simulink model "Model_plane5Old_vers"  (R2021a)
settings: Solver=VariableStepAuto  StartTime=0.0  StopTime=200  RelTol=1e-3
model workspace (MAT data in the model file):
  Alfa = [-2 4 10 16]
  Alfa_table = [-4 0 5 10 20]
  Alfa_y = [-4 6 8 9 10 12 14]
  Cxa_table = [0.03434  0.0358  0.04274; 0.02598  0.0252  0.0262; 0.04151  0.0505  0.0883; 0.122  0.1649  0.2341; 0.502  0.538  0.666]
  Cy_DB = [0.01242 0.01286 0.01457]
  Cy_fi = [0.00623 0.00643 0.00626]
  Cya = [-0.276  -0.33  -0.39; 0.859  0.991  0.82; 1.085  1.211  1.1; 1.2  1.275  1.031; 1.296  1.29  1.018; 1.45  1.178  1.043; 1.461  1.163  1.081]
  H = [339 3256 4060 8000 12000]
  H_table = [0 2000 4000 6000 8000 10000]
  M_C = [0.4 0.6 0.82]
  M_mz = [0.2 0.4 0.6 0.8]
  M_mz2 = [0.4 0.7 0.85]
  M_table = [0.4 0.7 0.82]
  M_y = [0.4 0.7 0.82]
  P = [50000 40000 32000 25600 20480]
  a_table = [340.3 339.5 338.8 338 337.2 336.4]
  mz_DB = [-0.035 -0.0358 -0.037 -0.0377]
  mz_alfa = [-0.0282 -0.0282 -0.0289 -0.0404]
  mz_alfa2 = [-8.163  -8.762  -9.714; -8.163  -8.762  -9.583; -7.975  -7.991  -7.868; -6.514  -6.413  -6.732]
  mz_fi = [-0.0695 -0.0714 -0.0739 -0.0832]
  mz_omz = [-23.768  -25.3  -28.284; -23.768  -25.3  -27.903; -23.222  -22.6  -23.32; -18.967  -18.52  -19.601]
  out = Simulink.SimulationOutput
  out.Data.tout = [0 1.67688873362e-06 9.33181354111e-06 4.76064375786e-05 0.000238979557766 0.0011958451587 0.00598017316339 0.0291858115735 0.107609227908 0.294605508218 0.534390352194 0.619831316604 ... (6422 elements, 6422x1)]
  out.Metadata = Simulink.SimulationMetadata
  out.Metadata.ModelInfo.ModelName = 'Model_plane2'
  out.Metadata.ModelInfo.ModelVersion = '1.11'
  out.Metadata.ModelInfo.ModelFilePath = 'C:\Users\Анастасия\Универ\Mathlab\Модель самолёта\Model_plane2.slx'
  out.Metadata.ModelInfo.UserID = 'Анастасия'
  out.Metadata.ModelInfo.MachineName = 'DESKTOP-OE36224'
  out.Metadata.ModelInfo.Platform = 'PCWIN64'
  out.Metadata.ModelInfo.ModelStructuralChecksum = [329193822; 1830100004; 2373400892; 4162968501]
  out.Metadata.ModelInfo.SimulationMode = 'normal'
  out.Metadata.ModelInfo.StartTime = 0
  out.Metadata.ModelInfo.StopTime = 100
  out.Metadata.ModelInfo.SolverInfo.Type = 'Variable-Step'
  out.Metadata.ModelInfo.SolverInfo.Solver = 'ode45'
  out.Metadata.ModelInfo.SolverInfo.MaxStepSize = 2
  out.Metadata.ModelInfo.SimulinkVersion.Name = 'Simulink'
  out.Metadata.ModelInfo.SimulinkVersion.Version = '24.1'
  out.Metadata.ModelInfo.SimulinkVersion.Release = '(R2024a)'
  out.Metadata.ModelInfo.SimulinkVersion.Date = '19-Nov-2023'
  out.Metadata.ModelInfo.LoggingInfo.LoggingToFile = 'off'
  out.Metadata.TimingInfo.WallClockTimestampStart = '2025-02-14 11:01:22'
  out.Metadata.TimingInfo.WallClockTimestampStop = '2025-02-14 11:01:24'
  out.Metadata.TimingInfo.InitializationElapsedWallTime = 1.1990057
  out.Metadata.TimingInfo.ExecutionElapsedWallTime = 1.0786509
  out.Metadata.TimingInfo.TerminationElapsedWallTime = 0.0112241
  out.Metadata.TimingInfo.TotalElapsedWallTime = 2.2888807
  out.Metadata.TimingInfo.ProfilerData = 'Profiler is not enabled'
  out.Metadata.ExecutionInfo.StopEvent = 'ReachedStopTime'
  out.Metadata.ExecutionInfo.StopEventSource = []
  out.Metadata.ExecutionInfo.StopEventDescription = 'Reached stop time of 100'
  out.Metadata.ExecutionInfo.ErrorDiagnostic = []
  out.Metadata.ExecutionInfo.WarningDiagnostics.Diagnostic = MSLDiagnostic
  out.Metadata.ExecutionInfo.WarningDiagnostics.Diagnostic.identifier = 'Simulink:blocks:DivideByZero'
  out.Metadata.ExecutionInfo.WarningDiagnostics.Diagnostic.message = 'Division by zero in ''<a href="matlab:open_and_hilite_hyperlink (''Model_plane2/Уравнения продольного движения в связанной системе координат/Блок расчёта угла атаки Alfa/Divide'',''error'')">Model_plane2/Уравнения продольного движения в связанной системе координат/Блок расчёта угла атаки Alfa/Divide</a>'''
  out.Metadata.ExecutionInfo.WarningDiagnostics.Diagnostic.paths = {'Model_plane2/Уравнения продольного движения в связанной системе координат/Блок расчёта угла атаки Alfa/Divide'}
  out.Metadata.ExecutionInfo.WarningDiagnostics.Diagnostic.arguments = {'Model_plane2/Уравнения продольного движения в связанной системе координат/Блок расчёта угла атаки Alfa/Divide'}
  out.Metadata.ExecutionInfo.WarningDiagnostics.Diagnostic.stack = struct([])
  out.Metadata.ExecutionInfo.WarningDiagnostics.Diagnostic.actionProp = '22 serialization::archive 19 0 0 0  0 1 0 0 1 1 0 0 0 0 0 1 47 SL_SERVICES:utils:EMBEDDED____ACTION____WRAPPER 2 2 0 0 183 0 109 97 116 108 97 98 58 83 105 109 117 108 105 110 107 46 83 117 112 112 114 101 115 115 101 100 68 105 97 103 110 111 115 116 105 99 40 123 39 77 111 100 101 108 95 112 108 97 110 101 50 47 1059 1088 1072 1074 1085 1077 1085 1080 1103 32 1087 1088 1086 1076 1086 1083 1100 1085 1086 1075 1086 32 1076 1074 1080 1078 1077 1085 1080 1103 32 1074 32 1089 1074 1103 1079 1072 1085 1085 1086 1081 32 1089 1080 1089 1090 1077 1084 1077 32 1082 1086 1086 1088 1076 1080 1085 1072 1090 47 1041 1083 1086 1082 32 1088 1072 1089 1095 1105 1090 1072 32 1091 1075 1083 1072 32 1072 1090 1072 1082 1080 32 65 108 102 97 47 68 105 118 105 100 101 39 125 44 39 83 105 109 117 108 105 110 107 58 98 108 111 99 107 115 58 68 105 118 105 100 101 66 121 90 101 114 111 39 41 59 2 0 0 1 6 0 0 0 0 0  1 0 0 0 0'
  out.Metadata.ExecutionInfo.WarningDiagnostics.Diagnostic.metaDataProp.UI = []
  out.Metadata.ExecutionInfo.WarningDiagnostics.Diagnostic.metaDataProp.STAGE = []
  out.Metadata.ExecutionInfo.WarningDiagnostics.Diagnostic.metaDataProp.CATEGORY = []
  out.Metadata.ExecutionInfo.WarningDiagnostics.Diagnostic.metaDataProp.COMPONENT = []
  out.Metadata.ExecutionInfo.WarningDiagnostics.Diagnostic.metaDataProp.MDL_NAME = []
  out.Metadata.ExecutionInfo.WarningDiagnostics.Diagnostic.metaDataProp.ACTION = '22 serialization::archive 19 0 0 0  0 1 0 0 1 1 0 0 0 0 0 1 47 SL_SERVICES:utils:EMBEDDED____ACTION____WRAPPER 2 2 0 0 183 0 109 97 116 108 97 98 58 83 105 109 117 108 105 110 107 46 83 117 112 112 114 101 115 115 101 100 68 105 97 103 110 111 115 116 105 99 40 123 39 77 111 100 101 108 95 112 108 97 110 101 50 47 1059 1088 1072 1074 1085 1077 1085 1080 1103 32 1087 1088 1086 1076 1086 1083 1100 1085 1086 1075 1086 32 1076 1074 1080 1078 1077 1085 1080 1103 32 1074 32 1089 1074 1103 1079 1072 1085 1085 1086 1081 32 1089 1080 1089 1090 1077 1084 1077 32 1082 1086 1086 1088 1076 1080 1085 1072 1090 47 1041 1083 1086 1082 32 1088 1072 1089 1095 1105 1090 1072 32 1091 1075 1083 1072 32 1072 1090 1072 1082 1080 32 65 108 102 97 47 68 105 118 105 100 101 39 125 44 39 83 105 109 117 108 105 110 107 58 98 108 111 99 107 115 58 68 105 118 105 100 101 66 121 90 101 114 111 39 41 59 2 0 0 1 6 0 0 0 0 0  1 0 0 0 0'
  out.Metadata.ExecutionInfo.WarningDiagnostics.Diagnostic.metaDataProp.DOC = []
  out.Metadata.ExecutionInfo.WarningDiagnostics.Diagnostic.metaDataProp.SUB_CATEGORY = []
  out.Metadata.ExecutionInfo.WarningDiagnostics.Diagnostic.metaDataProp.MSTACK_PRESERVE = []
  out.Metadata.ExecutionInfo.WarningDiagnostics.Diagnostic.metaDataProp.DOUBLE_ARGS = []
  out.Metadata.ExecutionInfo.WarningDiagnostics.Diagnostic.metaDataProp.USER_DATA = []
  out.Metadata.ExecutionInfo.WarningDiagnostics.Diagnostic.priority = 2
  out.Metadata.ExecutionInfo.WarningDiagnostics.SimulationPhase = 'Execution'
  out.Metadata.ExecutionInfo.WarningDiagnostics.SimulationTime = 0
  out.Metadata.AppInfo = struct()
  q_table = [1.225 1.0065 0.8194 0.6601 0.5258 0.4135]
libraries: simulink x1
settings Model: Creator=Анастасия  LastModifiedBy=Анастасия
settings DebuggingCC: UnconnectedInputMsg=none  UnconnectedOutputMsg=none  UnconnectedLineMsg=none
settings ModelReferenceCC: EnableRefExpFcnMdlSchedulingChecks=off
settings RTWCC: Description=Generic Real-Time Target  GPUComputeCapability=5.0  DLArmComputeVersion=20.02.1

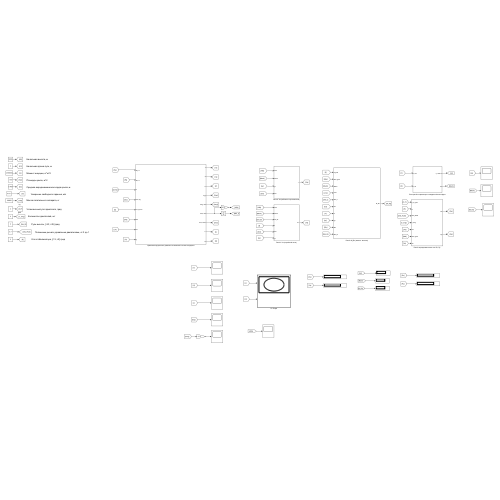
[thumbnail: Simulink's stored preview of the top-level diagram]
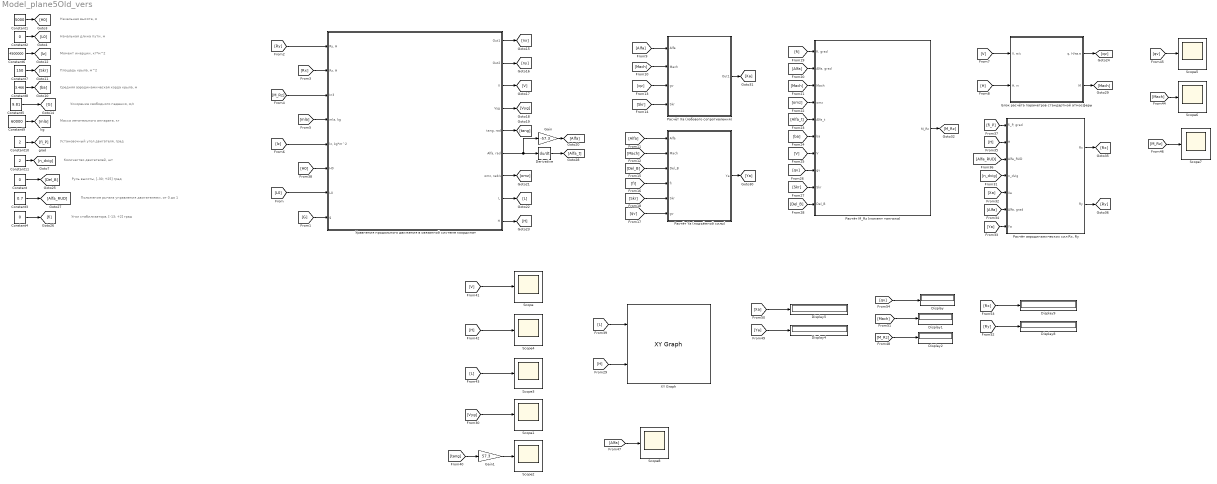
== system Model_plane5Old_vers ==
  note: Количество двигателей, шт
  note: Установочный угол двигателя, град
  note: Масса летательного аппарата, кг
  note: Средняя аэродинамическая хорда крыла, м
  note: Площадь крыла, м^2
  note: Момент инерции, кг*м^2
  note: Начальная длина пути, м
  note: Начальная высота, м
  note: Ускорение свободного падения, м/c
  note: Положение рычага управления двигателями, от 0 до 1
  note: Угол стабилизатора, [-13; +2] град
  note: Руль высоты, [-30; +25] град
  Constant : Constant  Value=0
  Constant1 : Constant  Value=5000
  Constant10 : Constant  Value=2
  Constant11 : Constant  Value=2
  Constant2 : Constant  Value=0
  Constant3 : Constant  Value=0.7
  Constant4 : Constant  Value=0
  Constant5 : Constant  Value=9.81
  Constant6 : Constant  Value=4500000
  Constant7 : Constant  Value=150
  Constant8 : Constant  Value=3.466
  Constant9 : Constant  Value=60000
  Derivative : Derivative
  Display{,1..2,4..5,8..9} (7 alike) : Display
  Gain : Gain  Gain=-57.3
  Gain1 : Gain  Gain=57.3
  Scope{,1..8} (9 alike) : Scope
  XY Graph : simulink/Sinks/XY Graph  xmin=-1  xmax=1  ymin=-1  ymax=1  st=-1
  Блок расчёта параметров стандартной атмосферы : Subsystem
  Расчёт M_Rz (момент тангажа) : Subsystem
  Расчёт Xa (лобового сопротивления) : Subsystem
  Расчёт Ya (подъёмной силы) : Subsystem
  "Расчёт аэродинамических сил Rx, Ry" : Subsystem
  Уравнения продольного движения в связанной системе координат : Subsystem
  wires:
  Constant1/1 -> [H0]
  Constant2/1 -> [L0]
  Constant6/1 -> [lz]
  Constant7/1 -> [Skr]
  Constant8/1 -> [ba]
  Constant9/1 -> [mla]
  Constant10/1 -> [fi_P]
  Constant11/1 -> [n_dvig]
  Constant5/1 -> [G]
  [Ry] -> Уравнения продольного движения в связанной системе координат/1("Ry, H")
  [Rx] -> Уравнения продольного движения в связанной системе координат/2("Rx, H")
  [M_Rz] -> Уравнения продольного движения в связанной системе координат/3(In3)
  [mla] -> Уравнения продольного движения в связанной системе координат/4("mla, kg")
  [lz] -> Уравнения продольного движения в связанной системе координат/5("lz, kg*m^2")
  Уравнения продольного движения в связанной системе координат/1(Out1) -> [nx]
  Уравнения продольного движения в связанной системе координат/2(Out2) -> [ny]
  Уравнения продольного движения в связанной системе координат/3(V) -> [V]
  Уравнения продольного движения в связанной системе координат/4(Vyg) -> [Vyg]
  Уравнения продольного движения в связанной системе координат/5("tang, rad") -> [tang]
  Уравнения продольного движения в связанной системе координат/6("Alfa, rad") -> Gain/1, Derivative/1
  Уравнения продольного движения в связанной системе координат/7("omz, rad/s") -> [omz]
  Уравнения продольного движения в связанной системе координат/8(L) -> [L]
  Уравнения продольного движения в связанной системе координат/9(H) -> [H]
  Derivative/1 -> [Alfa_t]
  [V] -> Блок расчёта параметров стандартной атмосферы/1("V, м/с")
  [H] -> Блок расчёта параметров стандартной атмосферы/2("H, м")
  Блок расчёта параметров стандартной атмосферы/1("q, Н/кв.м") -> [qv]
  Блок расчёта параметров стандартной атмосферы/2(М) -> [Mach]
  [Alfa] -> Расчёт Xa (лобового сопротивления)/1(Alfa)
  [Mach] -> Расчёт Xa (лобового сопротивления)/2(Mach)
  [Mach] -> Расчёт Ya (подъёмной силы)/2(Mach)
  [Alfa] -> Расчёт Ya (подъёмной силы)/1(Alfa)
  Расчёт Xa (лобового сопротивления)/1(Out1) -> [Xa]
  Расчёт Ya (подъёмной силы)/1(Ya) -> [Ya]
  [Skr] -> Расчёт Xa (лобового сопротивления)/4(Skr)
  [qv] -> Расчёт Xa (лобового сопротивления)/3(gv)
  [Del_B] -> Расчёт Ya (подъёмной силы)/3(Del_B)
  [fi] -> Расчёт Ya (подъёмной силы)/4(fi)
  [qv] -> Расчёт Ya (подъёмной силы)/6(gv)
  [Skr] -> Расчёт Ya (подъёмной силы)/5(Skr)
  Расчёт M_Rz (момент тангажа)/1(M_Rz) -> [M_Rz]
  [fi] -> Расчёт M_Rz (момент тангажа)/1("fi, grad")
  [Alfa] -> Расчёт M_Rz (момент тангажа)/2("Alfa, grad")
  [omz] -> Расчёт M_Rz (момент тангажа)/4(omz)
  [Mach] -> Расчёт M_Rz (момент тангажа)/3(Mach)
  [Alfa_t] -> Расчёт M_Rz (момент тангажа)/5(Alfa_t)
  [ba] -> Расчёт M_Rz (момент тангажа)/6(ba)
  [qv] -> Расчёт M_Rz (момент тангажа)/8(gv)
  [Del_B] -> Расчёт M_Rz (момент тангажа)/10(Del_B)
  [Skr] -> Расчёт M_Rz (момент тангажа)/9(Skr)
  [V] -> Расчёт M_Rz (момент тангажа)/7(V)
  "Расчёт аэродинамических сил Rx, Ry"/1(Rx) -> [Rx]
  "Расчёт аэродинамических сил Rx, Ry"/2(Ry) -> [Ry]
  [Alfa_RUD] -> "Расчёт аэродинамических сил Rx, Ry"/3(Alfa_RUD)
  [n_dvig] -> "Расчёт аэродинамических сил Rx, Ry"/4(n_dvig)
  [H] -> "Расчёт аэродинамических сил Rx, Ry"/2(H)
  [fi_P] -> "Расчёт аэродинамических сил Rx, Ry"/1("fi_P, grad")
  [H0] -> Уравнения продольного движения в связанной системе координат/6(H0)
  [L0] -> Уравнения продольного движения в связанной системе координат/7(L0)
  [G] -> Уравнения продольного движения в связанной системе координат/8(g)
  [V] -> Scope/1
  Constant4/1 -> [fi]
  Constant3/1 -> [Alfa_RUD]
  Constant/1 -> [Del_B]
  [H] -> Scope4/1
  [L] -> Scope3/1
  [Ya] -> "Расчёт аэродинамических сил Rx, Ry"/7(Ya)
  [Alfa] -> "Расчёт аэродинамических сил Rx, Ry"/6("Alfa, grad")
  [Xa] -> "Расчёт аэродинамических сил Rx, Ry"/5(Xa)
  [Vyg] -> Scope1/1
  [L] -> XY Graph/1
  [H] -> XY Graph/2
  [qv] -> Scope5/1
  [Mach] -> Scope6/1
  [M_Rz] -> Scope7/1
  [Alfa] -> Scope8/1
  [tang] -> Gain1/1
  Gain1/1 -> Scope2/1
  [Mach] -> Display1/1
  [M_Rz] -> Display2/1
  [Ry] -> Display8/1
  [Xa] -> Display5/1
  [Ya] -> Display4/1
  [Rx] -> Display9/1
  [qv] -> Display/1
  Gain/1 -> [Alfa]

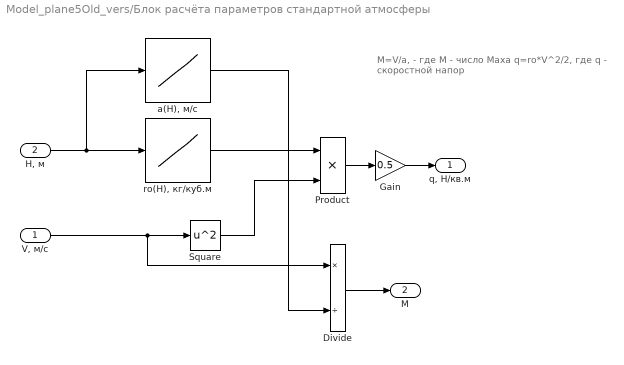
== system Model_plane5Old_vers/Блок расчёта параметров стандартной атмосферы ==
  note: M=V/a, - где М - число Маха
      | q=ro*V^2/2, где q - скоростной напор
  "V, м/с" : Inport
  "H, м" : Inport  Port=2
  Divide : Product  Inputs=*/
  Gain : Gain  Gain=0.5
  Product : Product
  Square : Math  Operator=square  SaturateOnIntegerOverflow=on
  "a(H), м/с" : Lookup_n-D  NumberOfTableDimensions=1  BreakpointsForDimension1=H_table  Table=a_table  InternalRulePriority=Speed  RndMeth=Simplest  InputSameDT=on
  "ro(H), кг/куб.м" : Lookup_n-D  NumberOfTableDimensions=1  BreakpointsForDimension1=H_table  Table=q_table  InternalRulePriority=Speed  RndMeth=Simplest  InputSameDT=on
  "q, Н/кв.м" : Outport
  М : Outport  Port=2
  wires:
  Gain/1 -> "q, Н/кв.м"/1
  "H, м"/1 -> "a(H), м/с"/1, "ro(H), кг/куб.м"/1
  Square/1 -> Product/2
  "V, м/с"/1 -> Square/1, Divide/1
  "ro(H), кг/куб.м"/1 -> Product/1
  "a(H), м/с"/1 -> Divide/2
  Product/1 -> Gain/1
  Divide/1 -> М/1

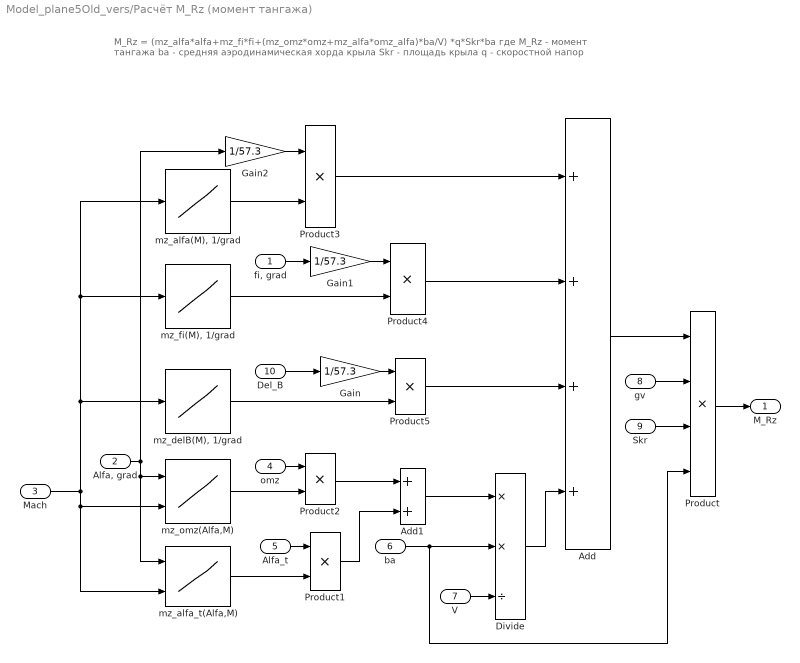
== system Model_plane5Old_vers/Расчёт M_Rz (момент тангажа) ==
  note: M_Rz = (mz_alfa*alfa+mz_fi*fi+(mz_omz*omz+mz_alfa*omz_alfa)*ba/V) *q*Skr*ba
      | где M_Rz - момент тангажа
      | ba - средняя аэродинамическая хорда крыла
      | Skr - площадь крыла
      | q - скоростной напор
  "fi, grad" : Inport
  "Alfa, grad" : Inport  Port=2
  Mach : Inport  Port=3
  omz : Inport  Port=4
  Alfa_t : Inport  Port=5
  ba : Inport  Port=6
  V : Inport  Port=7
  gv : Inport  Port=8
  Skr : Inport  Port=9
  Del_B : Inport  Port=10
  Add : Sum  Inputs=++++
  Add1 : Sum
  Divide : Product  Inputs=**/
  Gain : Gain  Gain=1/57.3
  Gain1 : Gain  Gain=1/57.3
  Gain2 : Gain  Gain=1/57.3
  Product : Product  Inputs=4
  Product{1..5} (5 alike) : Product
  "mz_alfa(M), 1/grad" : Lookup_n-D  NumberOfTableDimensions=1  BreakpointsForDimension1=M_mz  Table=mz_alfa  InternalRulePriority=Speed  RndMeth=Simplest  InputSameDT=on
  mz_alfa_t(Alfa,M) : Lookup_n-D  BreakpointsForDimension1=Alfa  BreakpointsForDimension2=M_mz2  Table=mz_alfa2  InternalRulePriority=Speed  RndMeth=Simplest  InputSameDT=on
      settings: InputPortMap=u0,u1
  "mz_delB(M), 1/grad" : Lookup_n-D  NumberOfTableDimensions=1  BreakpointsForDimension1=M_mz  Table=mz_DB  InternalRulePriority=Speed  RndMeth=Simplest  InputSameDT=on
  "mz_fi(M), 1/grad" : Lookup_n-D  NumberOfTableDimensions=1  BreakpointsForDimension1=M_mz  Table=mz_fi  InternalRulePriority=Speed  RndMeth=Simplest  InputSameDT=on
  mz_omz(Alfa,M) : Lookup_n-D  BreakpointsForDimension1=Alfa  BreakpointsForDimension2=M_mz2  Table=mz_omz  InternalRulePriority=Speed  RndMeth=Simplest  InputSameDT=on
      settings: InputPortMap=u0,u1
  M_Rz : Outport
  wires:
  Product/1 -> M_Rz/1
  ba/1 -> Product/4, Divide/2
  Skr/1 -> Product/3
  gv/1 -> Product/2
  Add/1 -> Product/1
  V/1 -> Divide/3
  Divide/1 -> Add/4
  Add1/1 -> Divide/1
  Product2/1 -> Add1/1
  Product1/1 -> Add1/2
  Alfa_t/1 -> Product1/1
  omz/1 -> Product2/1
  mz_omz(Alfa,M)/1 -> Product2/2
  mz_alfa_t(Alfa,M)/1 -> Product1/2
  Mach/1 -> mz_omz(Alfa,M)/2, mz_alfa_t(Alfa,M)/2, "mz_alfa(M), 1/grad"/1, "mz_fi(M), 1/grad"/1, "mz_delB(M), 1/grad"/1
  "mz_alfa(M), 1/grad"/1 -> Product3/2
  "mz_fi(M), 1/grad"/1 -> Product4/2
  "mz_delB(M), 1/grad"/1 -> Product5/2
  Product3/1 -> Add/1
  Product4/1 -> Add/2
  Product5/1 -> Add/3
  Del_B/1 -> Gain/1
  Gain/1 -> Product5/1
  "fi, grad"/1 -> Gain1/1
  Gain1/1 -> Product4/1
  "Alfa, grad"/1 -> Gain2/1, mz_omz(Alfa,M)/1, mz_alfa_t(Alfa,M)/1
  Gain2/1 -> Product3/1

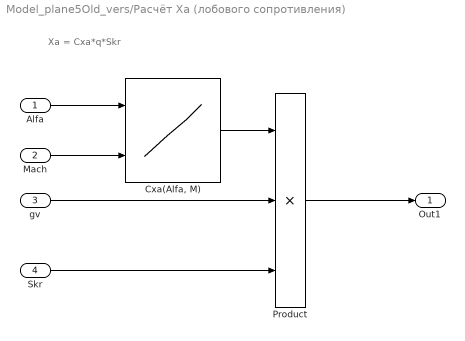
== system Model_plane5Old_vers/Расчёт Xa (лобового сопротивления) ==
  note: Xa = Cxa*q*Skr
  Alfa : Inport
  Mach : Inport  Port=2
  gv : Inport  Port=3
  Skr : Inport  Port=4
  "Cxa(Alfa, M)" : Lookup_n-D  BreakpointsForDimension1=Alfa_table  BreakpointsForDimension2=M_table  Table=Cxa_table  InternalRulePriority=Speed  RndMeth=Simplest  InputSameDT=on
      settings: InputPortMap=u0,u1
  Product : Product  Inputs=3
  Out1 : Outport
  wires:
  Alfa/1 -> "Cxa(Alfa, M)"/1
  Product/1 -> Out1/1
  Skr/1 -> Product/3
  gv/1 -> Product/2
  Mach/1 -> "Cxa(Alfa, M)"/2
  "Cxa(Alfa, M)"/1 -> Product/1

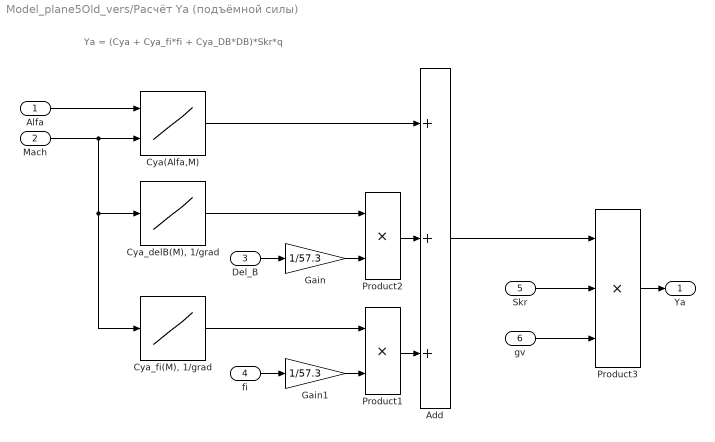
== system Model_plane5Old_vers/Расчёт Ya (подъёмной силы) ==
  note: Ya = (Cya + Cya_fi*fi + Cya_DB*DB)*Skr*q
  Alfa : Inport
  Mach : Inport  Port=2
  Del_B : Inport  Port=3
  fi : Inport  Port=4
  Skr : Inport  Port=5
  gv : Inport  Port=6
  Add : Sum  Inputs=+++
  Cya(Alfa,M) : Lookup_n-D  BreakpointsForDimension1=Alfa_y  BreakpointsForDimension2=M_y  Table=Cya  InternalRulePriority=Speed  RndMeth=Simplest  InputSameDT=on
      settings: InputPortMap=u0,u1
  "Cya_delB(M), 1/grad" : Lookup_n-D  NumberOfTableDimensions=1  BreakpointsForDimension1=M_C  Table=Cy_DB  InternalRulePriority=Speed  RndMeth=Simplest  InputSameDT=on
  "Cya_fi(M), 1/grad" : Lookup_n-D  NumberOfTableDimensions=1  BreakpointsForDimension1=M_C  Table=Cy_fi  InternalRulePriority=Speed  RndMeth=Simplest  InputSameDT=on
  Gain : Gain  Gain=1/57.3
  Gain1 : Gain  Gain=1/57.3
  Product1 : Product
  Product2 : Product
  Product3 : Product  Inputs=3
  Ya : Outport
  wires:
  Alfa/1 -> Cya(Alfa,M)/1
  gv/1 -> Product3/3
  Skr/1 -> Product3/2
  Product3/1 -> Ya/1
  "Cya_fi(M), 1/grad"/1 -> Product1/1
  "Cya_delB(M), 1/grad"/1 -> Product2/1
  Mach/1 -> "Cya_delB(M), 1/grad"/1, "Cya_fi(M), 1/grad"/1, Cya(Alfa,M)/2
  Cya(Alfa,M)/1 -> Add/1
  Product2/1 -> Add/2
  Product1/1 -> Add/3
  Add/1 -> Product3/1
  Del_B/1 -> Gain/1
  Gain/1 -> Product2/2
  fi/1 -> Gain1/1
  Gain1/1 -> Product1/2

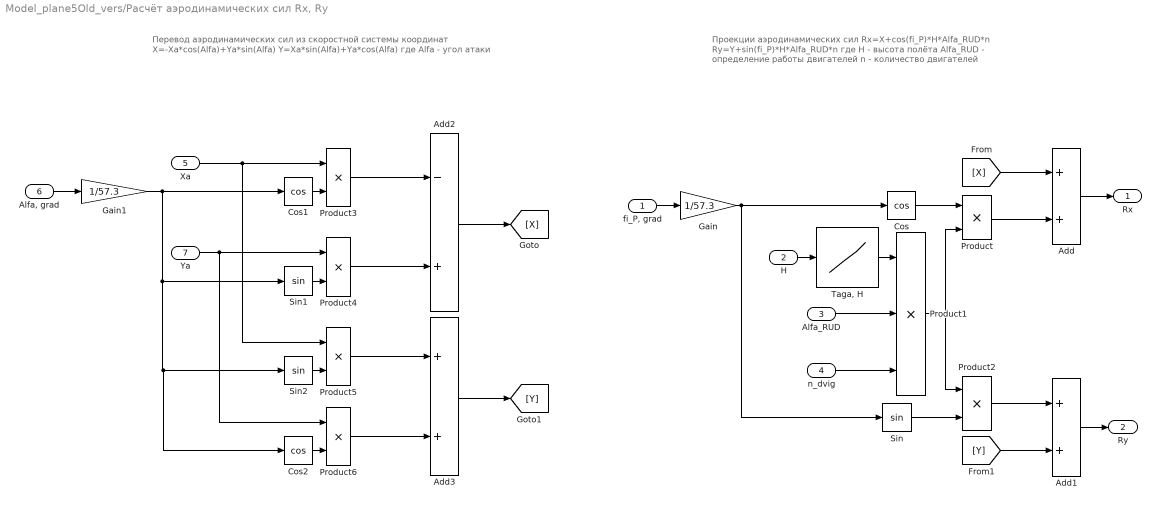
== system Model_plane5Old_vers/Расчёт аэродинамических сил Rx, Ry ==
  note: Проекции аэродинамических сил
      | Rx=X+cos(fi_P)*H*Alfa_RUD*n
      | Ry=Y+sin(fi_P)*H*Alfa_RUD*n
      | где Н - высота полёта
      | Alfa_RUD - определение работы двигателей
      | n - количество двигателей
  note: Перевод аэродинамических сил из скоростной системы координат
      | X=-Xa*cos(Alfa)+Ya*sin(Alfa)
      | Y=Xa*sin(Alfa)+Ya*cos(Alfa)
      | где Alfa - угол атаки
  "fi_P, grad" : Inport
  H : Inport  Port=2
  Alfa_RUD : Inport  Port=3
  n_dvig : Inport  Port=4
  Xa : Inport  Port=5
  "Alfa, grad" : Inport  Port=6
  Ya : Inport  Port=7
  Add : Sum
  Add1 : Sum
  Add2 : Sum  Inputs=-+
  Add3 : Sum
  Cos : Trigonometry  Operator=cos
  Cos1 : Trigonometry  Operator=cos
  Cos2 : Trigonometry  Operator=cos
  Gain : Gain  Gain=1/57.3
  Gain1 : Gain  Gain=1/57.3
  Product{,2..6} (6 alike) : Product
  Product1 : Product  Inputs=3
  Sin : Trigonometry
  Sin1 : Trigonometry
  Sin2 : Trigonometry
  "Taga, H" : Lookup_n-D  NumberOfTableDimensions=1  BreakpointsForDimension1=H  Table=P  InternalRulePriority=Speed  RndMeth=Simplest  InputSameDT=on
  Rx : Outport
  Ry : Outport  Port=2
  wires:
  [X] -> Add/1
  Product/1 -> Add/2
  Cos/1 -> Product/1
  Gain/1 -> Sin/1, Cos/1
  "fi_P, grad"/1 -> Gain/1
  "Taga, H"/1 -> Product1/1
  Alfa_RUD/1 -> Product1/2
  n_dvig/1 -> Product1/3
  H/1 -> "Taga, H"/1
  Product1/1 -> Product/2, Product2/1
  Sin/1 -> Product2/2
  Add/1 -> Rx/1
  Product2/1 -> Add1/1
  [Y] -> Add1/2
  Add1/1 -> Ry/1
  Add3/1 -> [Y]
  Add2/1 -> [X]
  Sin2/1 -> Product5/2
  Gain1/1 -> Cos2/1, Sin2/1, Sin1/1, Cos1/1
  Product3/1 -> Add2/1
  Product6/1 -> Add3/2
  Cos2/1 -> Product6/2
  Product5/1 -> Add3/1
  Product4/1 -> Add2/2
  "Alfa, grad"/1 -> Gain1/1
  Cos1/1 -> Product3/2
  Sin1/1 -> Product4/2
  Ya/1 -> Product6/1, Product4/1
  Xa/1 -> Product5/1, Product3/1

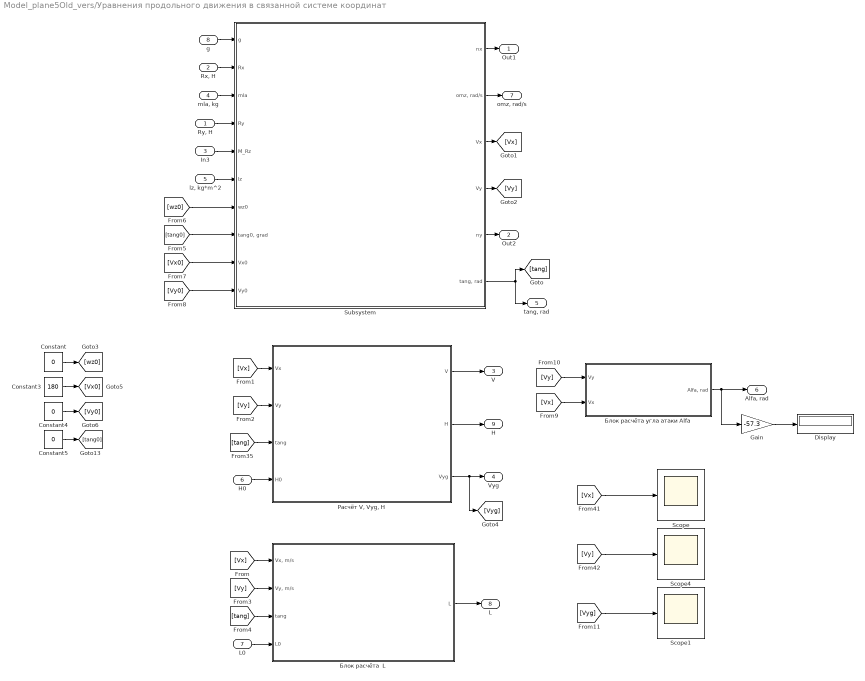
== system Model_plane5Old_vers/Уравнения продольного движения в связанной системе координат ==
  "Ry, H" : Inport
  "Rx, H" : Inport  Port=2
  In3 : Inport  Port=3
  "mla, kg" : Inport  Port=4
  "lz, kg*m^2" : Inport  Port=5
  H0 : Inport  Port=6
  L0 : Inport  Port=7
  g : Inport  Port=8
  Constant : Constant  Value=0
  Constant3 : Constant  Value=180
  Constant4 : Constant  Value=0
  Constant5 : Constant  Value=0
  Display : Display
  Gain : Gain  Gain=-57.3
  Scope : Scope
  Scope1 : Scope
  Scope4 : Scope
  Subsystem : Subsystem
  Блок расчёта  L : Subsystem
  Блок расчёта угла атаки Alfa : Subsystem
  "Расчёт V, Vyg, H" : Subsystem
  Out1 : Outport
  Out2 : Outport  Port=2
  V : Outport  Port=3
  Vyg : Outport  Port=4
  "tang, rad" : Outport  Port=5
  "Alfa, rad" : Outport  Port=6
  "omz, rad/s" : Outport  Port=7
  L : Outport  Port=8
  H : Outport  Port=9
  wires:
  [tang] -> "Расчёт V, Vyg, H"/3(tang)
  "Расчёт V, Vyg, H"/2(H) -> H/1
  "Расчёт V, Vyg, H"/3(Vyg) -> [Vyg], Vyg/1
  "Расчёт V, Vyg, H"/1(V) -> V/1
  H0/1 -> "Расчёт V, Vyg, H"/4(H0)
  Блок расчёта  L/1(L) -> L/1
  Subsystem/1(nx) -> Out1/1
  Subsystem/5(ny) -> Out2/1
  Subsystem/6("tang, rad") -> "tang, rad"/1, [tang]
  [Vx] -> "Расчёт V, Vyg, H"/1(Vx)
  [Vy] -> "Расчёт V, Vyg, H"/2(Vy)
  Subsystem/3(Vx) -> [Vx]
  Subsystem/4(Vy) -> [Vy]
  Subsystem/2("omz, rad/s") -> "omz, rad/s"/1
  [Vx] -> Блок расчёта  L/1("Vx, m/s")
  [Vy] -> Блок расчёта  L/2("Vy, m/s")
  [tang] -> Блок расчёта  L/3(tang)
  L0/1 -> Блок расчёта  L/4(L0)
  g/1 -> Subsystem/1(g)
  "Rx, H"/1 -> Subsystem/2(Rx)
  "Ry, H"/1 -> Subsystem/4(Ry)
  In3/1 -> Subsystem/5(M_Rz)
  "lz, kg*m^2"/1 -> Subsystem/6(lz)
  Constant5/1 -> [tang0]
  Constant4/1 -> [Vy0]
  Constant3/1 -> [Vx0]
  Constant/1 -> [wz0]
  [tang0] -> Subsystem/8("tang0, grad")
  [wz0] -> Subsystem/7(wz0)
  [Vx0] -> Subsystem/9(Vx0)
  [Vy0] -> Subsystem/10(Vy0)
  "mla, kg"/1 -> Subsystem/3(mla)
  Блок расчёта угла атаки Alfa/1("Alfa, rad") -> Gain/1, "Alfa, rad"/1
  [Vy] -> Scope4/1
  [Vx] -> Scope/1
  [Vyg] -> Scope1/1
  [Vx] -> Блок расчёта угла атаки Alfa/2(Vx)
  [Vy] -> Блок расчёта угла атаки Alfa/1(Vy)
  Gain/1 -> Display/1

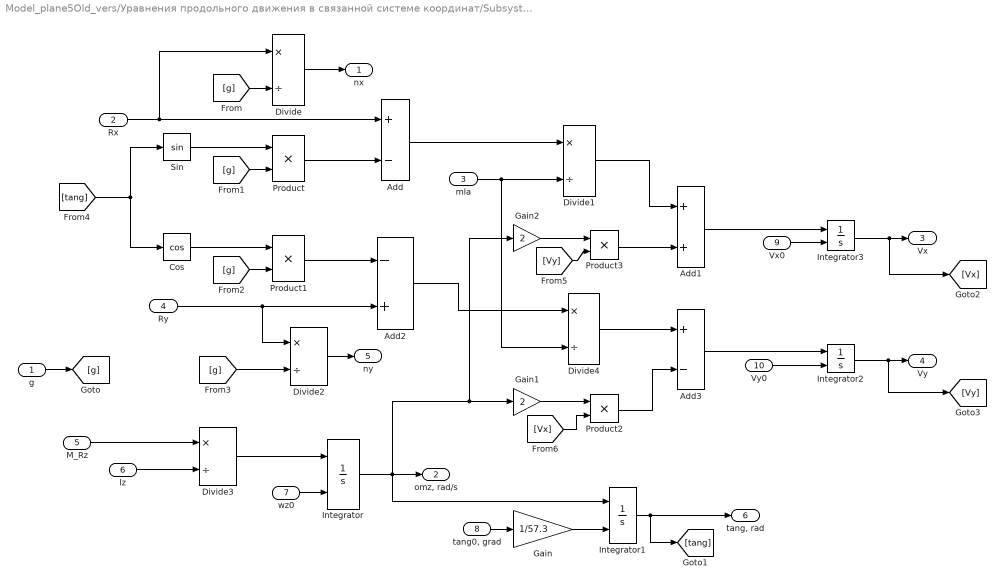
== system Model_plane5Old_vers/Уравнения продольного движения в связанной системе координат/Subsystem ==
  g : Inport
  Rx : Inport  Port=2
  mla : Inport  Port=3
  Ry : Inport  Port=4
  M_Rz : Inport  Port=5
  lz : Inport  Port=6
  wz0 : Inport  Port=7
  "tang0, grad" : Inport  Port=8
  Vx0 : Inport  Port=9
  Vy0 : Inport  Port=10
  Add : Sum  Inputs=+-
  Add1 : Sum
  Add2 : Sum  Inputs=-+
  Add3 : Sum  Inputs=+-
  Cos : Trigonometry  Operator=cos
  Divide{,1..4} (5 alike) : Product  Inputs=*/
  Gain : Gain  Gain=1/57.3
  Gain1 : Gain  Gain=2
  Gain2 : Gain  Gain=2
  Integrator{,1..3} (4 alike) : Integrator  InitialConditionSource=external
  Product{,1..3} (4 alike) : Product
  Sin : Trigonometry
  nx : Outport
  "omz, rad/s" : Outport  Port=2
  Vx : Outport  Port=3
  Vy : Outport  Port=4
  ny : Outport  Port=5
  "tang, rad" : Outport  Port=6
  wires:
  g/1 -> [g]
  Rx/1 -> Divide/1, Add/1
  Product/1 -> Add/2
  [g] -> Divide/2
  [g] -> Product/2
  Sin/1 -> Product/1
  [tang] -> Sin/1, Cos/1
  Divide/1 -> nx/1
  Add/1 -> Divide1/1
  mla/1 -> Divide4/2, Divide1/2
  Cos/1 -> Product1/1
  [g] -> Product1/2
  Product1/1 -> Add2/1
  Ry/1 -> Divide2/1, Add2/2
  [g] -> Divide2/2
  Divide2/1 -> ny/1
  M_Rz/1 -> Divide3/1
  lz/1 -> Divide3/2
  wz0/1 -> Integrator/2
  Divide3/1 -> Integrator/1
  Integrator/1 -> Integrator1/1, Gain2/1, Gain1/1, "omz, rad/s"/1
  Add2/1 -> Divide4/1
  Divide4/1 -> Add3/1
  Product2/1 -> Add3/2
  "tang0, grad"/1 -> Gain/1
  Gain/1 -> Integrator1/2
  Add3/1 -> Integrator2/1
  Add1/1 -> Integrator3/1
  Divide1/1 -> Add1/1
  Product3/1 -> Add1/2
  Integrator3/1 -> Vx/1, [Vx]
  Integrator2/1 -> [Vy], Vy/1
  Integrator1/1 -> [tang], "tang, rad"/1
  [Vy] -> Product3/2
  [Vx] -> Product2/2
  Vx0/1 -> Integrator3/2
  Vy0/1 -> Integrator2/2
  Gain1/1 -> Product2/1
  Gain2/1 -> Product3/1

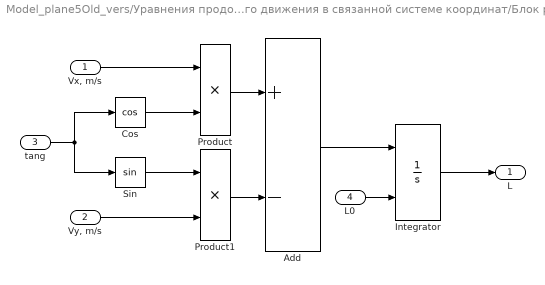
== system Model_plane5Old_vers/Уравнения продольного движения в связанной системе координат/Блок расчёта  L ==
  "Vx, m/s" : Inport
  "Vy, m/s" : Inport  Port=2
  tang : Inport  Port=3
  L0 : Inport  Port=4
  Add : Sum  Inputs=+-
  Cos : Trigonometry  Operator=cos
  Integrator : Integrator  InitialConditionSource=external
  Product : Product
  Product1 : Product
  Sin : Trigonometry
  L : Outport
  wires:
  "Vx, m/s"/1 -> Product/1
  tang/1 -> Sin/1, Cos/1
  Cos/1 -> Product/2
  Sin/1 -> Product1/1
  "Vy, m/s"/1 -> Product1/2
  Product/1 -> Add/1
  Product1/1 -> Add/2
  L0/1 -> Integrator/2
  Add/1 -> Integrator/1
  Integrator/1 -> L/1

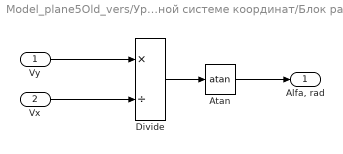
== system Model_plane5Old_vers/Уравнения продольного движения в связанной системе координат/Блок расчёта угла атаки Alfa ==
  Vy : Inport
  Vx : Inport  Port=2
  Atan : Trigonometry  Operator=atan
  Divide : Product  Inputs=*/
  "Alfa, rad" : Outport
  wires:
  Vy/1 -> Divide/1
  Vx/1 -> Divide/2
  Divide/1 -> Atan/1
  Atan/1 -> "Alfa, rad"/1

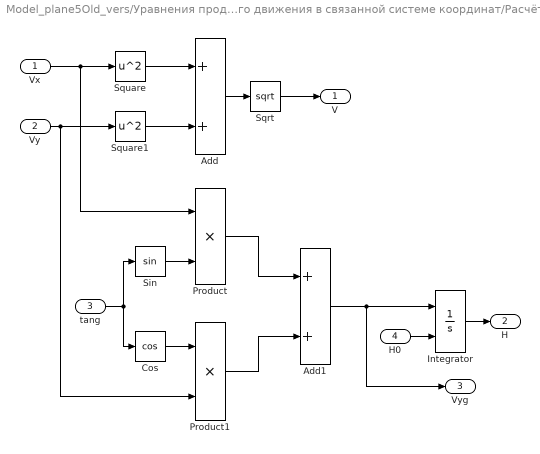
== system Model_plane5Old_vers/Уравнения продольного движения в связанной системе координат/Расчёт V, Vyg, H ==
  Vx : Inport
  Vy : Inport  Port=2
  tang : Inport  Port=3
  H0 : Inport  Port=4
  Add : Sum
  Add1 : Sum
  Cos : Trigonometry  Operator=cos
  Integrator : Integrator  InitialConditionSource=external
  Product : Product
  Product1 : Product
  Sin : Trigonometry
  Sqrt : Sqrt  IntermediateResultsDataTypeStr=double  SaturateOnIntegerOverflow=on
  Square : Math  Operator=square  SaturateOnIntegerOverflow=on
  Square1 : Math  Operator=square  SaturateOnIntegerOverflow=on
  V : Outport
  H : Outport  Port=2
  Vyg : Outport  Port=3
  wires:
  Vx/1 -> Square/1, Product/1
  Vy/1 -> Square1/1, Product1/2
  Square/1 -> Add/1
  Square1/1 -> Add/2
  Add/1 -> Sqrt/1
  Sqrt/1 -> V/1
  Cos/1 -> Product1/1
  Sin/1 -> Product/2
  tang/1 -> Cos/1, Sin/1
  Product/1 -> Add1/1
  Product1/1 -> Add1/2
  H0/1 -> Integrator/2
  Add1/1 -> Vyg/1, Integrator/1
  Integrator/1 -> H/1
